simulink model "bloques_temperatura"  (R2019a)
settings: Solver=VariableStepAuto  StartTime=0.0  StopTime=7000  RelTol=1e-3
values from neighbouring files (symbols this model uses):
  A = [-K1-K2,K2,0; K3, -K3-K4, K4;0,K5,-K5]    [params.m]
  B = [K0; 0;0]    [params.m]
  E = [K1*T0;0;0]    [params.m]
  x0 = [20,20,20]    [params.m]
settings Model: Creator=Dell  LastModifiedBy=pabli
settings DataIOCC: ReturnWorkspaceOutputs=off
settings DebuggingCC: PregeneratedLibrarySubsystemCodeDiagnostic=none  ArithmeticOperatorsInVariantConditions=warning
settings SFSimCC: SimUseLocalCustomCode=off
settings RTWCC: RTWUseLocalCustomCode=off

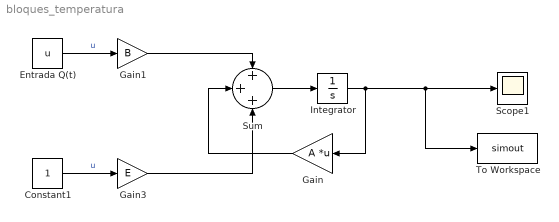
== system bloques_temperatura ==
  Constant1 : Constant
  Entrada Q(t) : Constant  Value=u
  Gain : Gain  Gain=A  Multiplication=Matrix(K*u)
  Gain1 : Gain  Gain=B
  Gain3 : Gain  Gain=E
  Integrator : Integrator  InitialCondition=x0'
  Scope1 : Scope
  Sum : Sum  Inputs=+++
  To Workspace : ToWorkspace  VariableName=simout  SampleTime=-1
  wires:
  Entrada Q(t)/1 -> Gain1/1  "u"
  Gain1/1 -> Sum/1
  Integrator/1 -> To Workspace/1, Scope1/1, Gain/1
  Gain/1 -> Sum/2
  Sum/1 -> Integrator/1
  Gain3/1 -> Sum/3
  Constant1/1 -> Gain3/1  "u"
